simulink library "family_19_variant_1_robot_drivers"  (R2014b)
settings: Solver=ode45  StartTime=0.0  StopTime=10.0  FixedStep=0.01  RelTol=1e-3
PreLoadFcn:
  | addLibrariesInPath('arduino')
  | addLibrariesInPath('rpi')
settings Model: Creator=odufour  LastModifiedBy=odufour

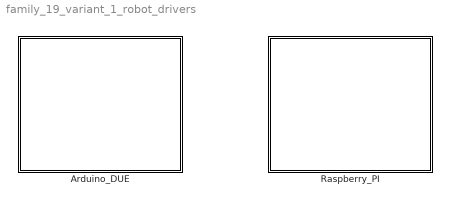
== system family_19_variant_1_robot_drivers ==
  Arduino_DUE : Subsystem
  Raspberry_PI : Subsystem

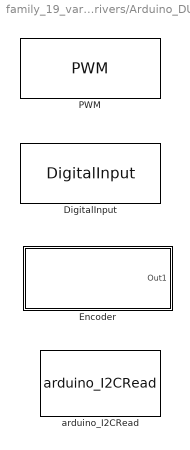
== system family_19_variant_1_robot_drivers/Arduino_DUE ==
  DigitalInput : S-Function  FunctionName=DigitalInput  Parameters=pinNumber, isPullUp  EnableBusSupport=off  mask(Arduino Digital Input){pinNumber=0, isPullUp=on}
      mask prompts: pinNumber "Pin Number"; isPullUp "Enable Pull Up"
      mask help:
      | Get the logical value of a specified digital input pin.
      |
      | Enter the number of the digital input pin (0-53 for Arduino Due). Do not assign the same pin number to multiple blocks within a model.
      mask init:
      | % Make sure that data type of pinNumber is UINT8
      | pinNumber = uint8(pinNumber);
      | 
      | % Make sure that data type of isPullUp is UINT8
      | isPullUp = uint8(isPullUp);
      mask Display: disp(sprintf('Arduino Digital Input\nPin n°%d',pinNumber))
  Encoder : Subsystem  mask{pinA=18, pinB=19}
      mask prompts: pinA "Pin A"; pinB "Pin B"
      mask Display: disp('Arduino Encoder')
  PWM : S-Function  FunctionName=PWM  Parameters=pinNumber  EnableBusSupport=off  mask(Arduino PWM){pinNumber=2}
      mask prompts: pinNumber "Pin Number"
      mask help:
      | Generate square waveform on the specified analog output pin. The block input controls the duty cycle of the square waveform. An input value of 0 produces a 0 percent duty cycle, and an input value of 255 produces a 100 percent duty cycle. The frequency of the waveform is constant at approximately 490 Hz.
      |
      | Enter the number of the analog output pin (2-13 for Arduino Due). Do not assign the same pin number to multiple blocks within a model.
      mask init:
      | % Make sure that pinNumber is an INT32
      | pinNumber = int32(pinNumber);
      mask Display: disp(sprintf('Arduino PWM\nPin n°%d',pinNumber))
  arduino_I2CRead : S-Function  FunctionName=arduino_I2CRead  Parameters=uint8(buffer_size)  EnableBusSupport=off  mask(I2C Read for Arduino Due){buffer_size=12}
      mask prompts: buffer_size "Buffer size"
      mask help:
      | Connect to I2C bus as a slave with address 0x12
      | Set the maximal size for data to receive with this block as buffer size

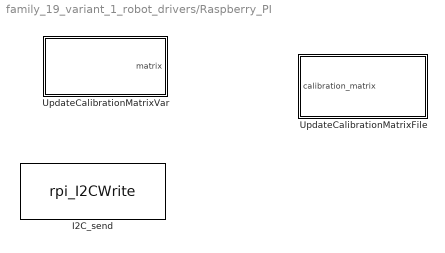
== system family_19_variant_1_robot_drivers/Raspberry_PI ==
  I2C_send : S-Function  FunctionName=rpi_I2CWrite  EnableBusSupport=off  mask(Send I2C){}
      mask help: Send input array of UINT8 through I2C channel
      mask Display: disp('Send I2C')
  UpdateCalibrationMatrixFile : Subsystem  mask(Write calibration matrix){filename='calibration.txt'}
      mask prompts: filename "Calibration file name"
      mask help: Write calibration matrix (input signal) in a text file named calibration.txt
      mask init:
      | filename = [uint8(filename), uint8(0)];
  UpdateCalibrationMatrixVar : Subsystem  mask(Read calibration matrix){dim=[3,3], filename='calibration.txt'}
      mask prompts: dim "Output dimension"; filename "Calibration file name"
      mask help:
      | Read calibration matrix from file calibration.txt
      | Output is an array of UINT8
      mask init:
      | filename = [uint8(filename),uint8(0)];
      | size = prod(dim);

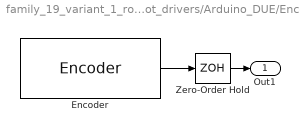
== system family_19_variant_1_robot_drivers/Arduino_DUE/Encoder ==
  Encoder : S-Function  FunctionName=Encoder  Parameters=pinA,pinB  EnableBusSupport=off  mask(Arduino Encoder){pinA=pinA, pinB=pinB}
      mask prompts: pinA "Pin A"; pinB "Pin B"
      mask init:
      | pinA = uint8(pinA);
      | pinB = uint8(pinB);
      mask Display: disp('Arduino Encoder')
  Zero-Order Hold : ZeroOrderHold  SampleTime=-1
  Out1 : Outport
  wires:
  Zero-Order Hold/1 -> Out1/1
  Encoder/1 -> Zero-Order Hold/1

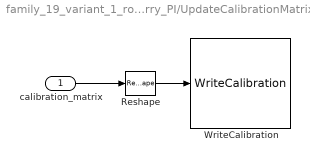
== system family_19_variant_1_robot_drivers/Raspberry_PI/UpdateCalibrationMatrixFile ==
  calibration_matrix : Inport
  Reshape : Reshape
  WriteCalibration : S-Function  FunctionName=WriteCalibration  Parameters=filename  EnableBusSupport=off
  wires:
  calibration_matrix/1 -> Reshape/1
  Reshape/1 -> WriteCalibration/1

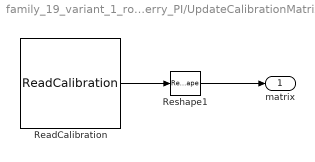
== system family_19_variant_1_robot_drivers/Raspberry_PI/UpdateCalibrationMatrixVar ==
  ReadCalibration : S-Function  FunctionName=ReadCalibration  Parameters=filename,size  EnableBusSupport=off
  Reshape1 : Reshape  OutputDimensionality=Customize  OutputDimensions=dim
  matrix : Outport
  wires:
  Reshape1/1 -> matrix/1
  ReadCalibration/1 -> Reshape1/1
